simulink model "logo_IO_task"  (Simulink 3.00)
libraries: mathlib x8, lib x2

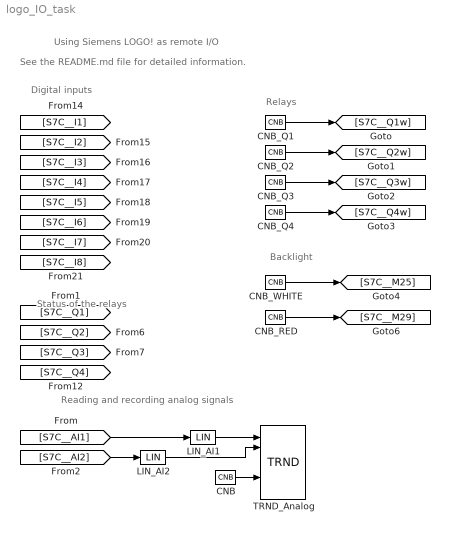
== system logo_IO_task ==
  note: Reading and recording analog signals
  note: Digital inputs
  note: Status of the relays
  note: Relays
  note: Backlight
  note: Using Siemens LOGO! as remote I/O
  note: See the README.md file for detailed information.
  CNB : lib/CNB  YCN=on
  CNB_Q1 : mathlib/CNB  YCN=on
  CNB_Q2 : mathlib/CNB  YCN=off
  CNB_Q3 : mathlib/CNB  YCN=on
  CNB_Q4 : mathlib/CNB  YCN=off
  CNB_RED : mathlib/CNB  YCN=off
  CNB_WHITE : mathlib/CNB  YCN=on
  LIN_AI1 : mathlib/LIN  u1=0  y1=0  u2=1000  y2=10
  LIN_AI2 : mathlib/LIN  u1=0  y1=0  u2=1000  y2=10
  TRND_Analog : lib/TRND  n=2  l=9000  btype=8: Double  ptype1=1: Store  ptype2=1: Store  ptype3=1: Store  ptype4=1: Store  pfac=1  afac=0  arc=0  id=2  Title=Analog signals  timesrc=1
  wires:
  CNB/1 -> TRND_Analog/5
  CNB_Q1/1 -> [S7C__Q1w]
  CNB_Q2/1 -> [S7C__Q2w]
  CNB_Q3/1 -> [S7C__Q3w]
  CNB_Q4/1 -> [S7C__Q4w]
  CNB_RED/1 -> [S7C__M29]
  CNB_WHITE/1 -> [S7C__M25]
  [S7C__AI1] -> LIN_AI1/1
  [S7C__AI2] -> LIN_AI2/1
  LIN_AI1/1 -> TRND_Analog/1
  LIN_AI2/1 -> TRND_Analog/2
